simulink model "DCDC_Buck"  (R2021b)
settings: Solver=VariableStepAuto  StartTime=0.0  StopTime=10.0  RelTol=1e-3
model workspace (MAT data in the model file):
  VSF = 0.439
undefined symbols (not defined in the file): FPWM, Gi, TBPRD, Tpwm, Ts
libraries: fl_lib x24, nesl_utility x6, ee_lib x3, tiiqmathlib x2, simulink x2
settings Model: Creator=win  LastModifiedBy=win

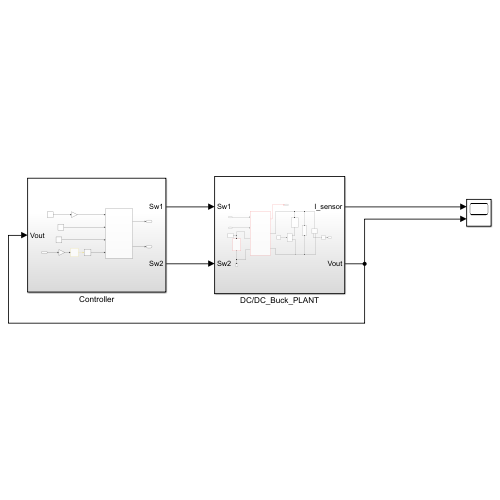
[thumbnail: Simulink's stored preview of the top-level diagram]
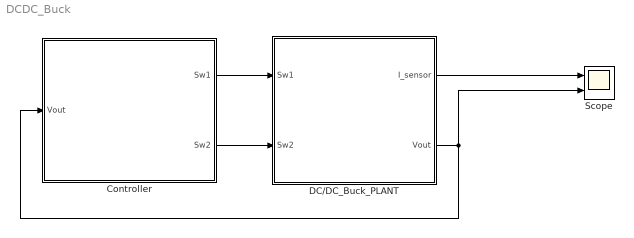
== system DCDC_Buck ==
  Controller : Subsystem
  DC/DC_Buck_PLANT : Subsystem
  Scope : Scope  NumInputPorts=2
  wires:
  Controller/1(Sw1) -> DC/DC_Buck_PLANT/1(Sw1)
  Controller/2(Sw2) -> DC/DC_Buck_PLANT/2(Sw2)
  DC/DC_Buck_PLANT/2(Vout) -> Controller/1(Vout), Scope/2
  DC/DC_Buck_PLANT/1(I_sensor) -> Scope/1

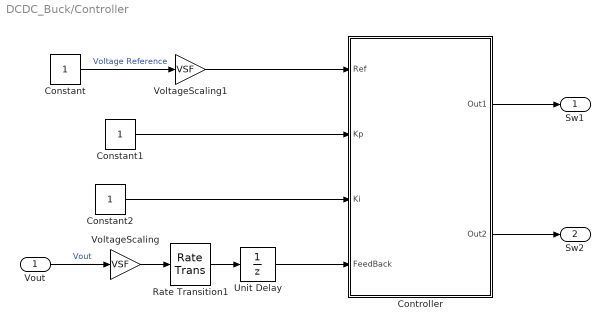
== system DCDC_Buck/Controller ==
  Vout : Inport
  Constant : Constant
  Constant1 : Constant
  Constant2 : Constant
  Controller : Subsystem
  Rate Transition1 : RateTransition  Integrity=off  Deterministic=off  OutPortSampleTime=Tcont
  Unit Delay : UnitDelay  SampleTime=-1  HasFrameUpgradeWarning=on
  VoltageScaling : Gain  Gain=VSF
  VoltageScaling1 : Gain  Gain=VSF
  Sw1 : Outport
  Sw2 : Outport  Port=2
  wires:
  Vout/1 -> VoltageScaling/1  "Vout"
  VoltageScaling/1 -> Rate Transition1/1
  Rate Transition1/1 -> Unit Delay/1
  Unit Delay/1 -> Controller/4(FeedBack)
  Constant/1 -> VoltageScaling1/1  "Voltage Reference"
  VoltageScaling1/1 -> Controller/1(Ref)
  Constant1/1 -> Controller/2(Kp)
  Constant2/1 -> Controller/3(Ki)
  Controller/1(Out1) -> Sw1/1
  Controller/2(Out2) -> Sw2/1

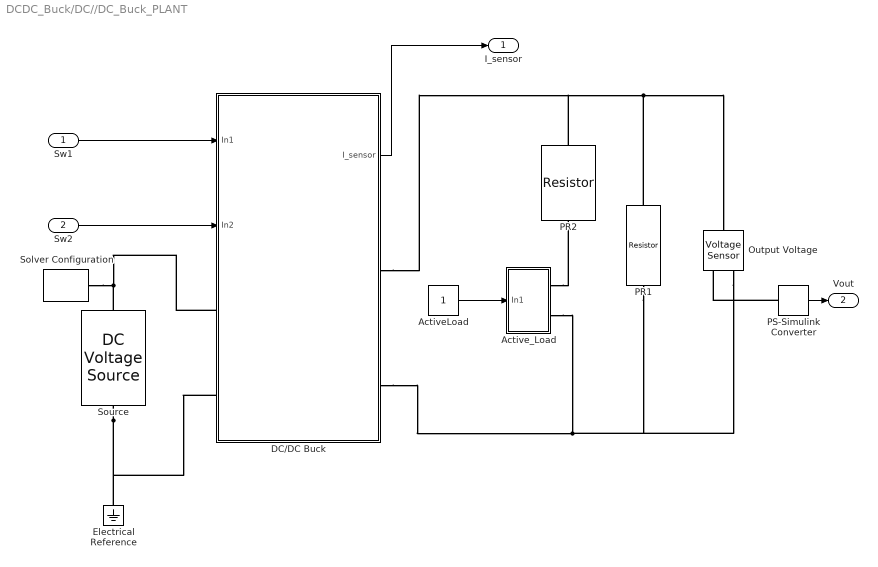
== system DCDC_Buck/DC//DC_Buck_PLANT ==
  Sw1 : Inport
  Sw2 : Inport  Port=2
  ActiveLoad : Constant
  Active_Load : Subsystem
  DC/DC Buck : Subsystem
  Electrical Reference : fl_lib/Electrical/Electrical Elements/Electrical Reference
  Output Voltage : fl_lib/Electrical/Electrical Sensors/Voltage Sensor  Priority=0
  PR1 : fl_lib/Electrical/Electrical Elements/Resistor  R=7.5 Ohm  i_specify=off  i_priority=None  i=0 A  i_nominal_specify=off  i_nominal_unit=A  i_nominal_value=1  v_specify=off  v_priority=None  v=0 V  v_nominal_specify=off  v_nominal_unit=V  v_nominal_value=1
  PR2 : fl_lib/Electrical/Electrical Elements/Resistor  R=2 Ohm  i_specify=off  i_priority=None  i=0 A  i_nominal_specify=off  i_nominal_unit=A  i_nominal_value=1  v_specify=off  v_priority=None  v=0 V  v_nominal_specify=off  v_nominal_unit=V  v_nominal_value=1
  PS-Simulink Converter : nesl_utility/PS-Simulink Converter  Priority=2  PhysicalDomain=network_engine_domain  SubClassName=ps_output  LeftPortType=input  RightPortType=output  PseudoPeriodic=off  Frequencies=[]  Unit=1  AffineConversion=off
      settings: SourceProductBaseCode=PW,SS
  Solver Configuration : nesl_utility/Solver Configuration  PhysicalDomain=network_engine_domain  SubClassName=solver  LeftPortType=input  RightPortType=generic  Tones=[]  Harmonics=[]  SimulateNoise=off  Profile=off  UseLocalSampling=off  EnableSwitchedLinearOptims=on  FrequencyDomain=off  UseCCode=off  RelTol=0.001  AbsTol=1e-06  MinStep=1e-09  ToWorkspace=off  RevertToSquareIcSolve=off  NumHomotopyIterations=100  PhasorMode=off  PhasorModeNumHarmonics=1  DoDC=off  ResidualTolerance=1e-08  UseLocalSolver=off  LocalSolverChoice=NE_TRAPEZOIDAL_ADVANCER  LocalSolverSampleTime=Ts/10  DoFixedCost=off  MaxNonlinIter=3  MaxModeIter=2  ComputeImpulses=off  ImpulseIterations=2  LinearAlgebra=Sparse  EquationFormulation=NE_TIME_EF  DelaysMemoryBudget=1024  AutomaticFiltering=on  FilteringTimeConstant=0.001  PartitionStorageMethod=AS_NEEDED  PartitionMemoryBudget=1024  PartitionMethod=FAST
      settings: SourceProductBaseCode=PW,SS
  Source : fl_lib/Electrical/Electrical Sources/DC Voltage Source  v0=9 V
  I_sensor : Outport  VectorParamsAs1DForOutWhenUnconnected=off
  Vout : Outport  Port=2  VectorParamsAs1DForOutWhenUnconnected=off
  wires:
  DC/DC Buck/1(I_sensor) -> I_sensor/1
  Sw2/1 -> DC/DC Buck/2(In2)
  Sw1/1 -> DC/DC Buck/1(In1)
  PS-Simulink Converter/1 -> Vout/1
  ActiveLoad/1 -> Active_Load/1(In1)
  connections:
  PS-Simulink Converter/LConn1 -- Output Voltage/RConn1
  Active_Load/RConn2 -- DC/DC Buck/RConn2 -- PR1/RConn1 -- Output Voltage/RConn2
  PR1/LConn1 -- Output Voltage/LConn1 -- DC/DC Buck/RConn1 -- PR2/LConn1
  Source/RConn1 -- DC/DC Buck/LConn2 -- Electrical Reference/LConn1
  Active_Load/RConn1 -- PR2/RConn1
  Solver Configuration/RConn1 -- DC/DC Buck/LConn1 -- Source/LConn1

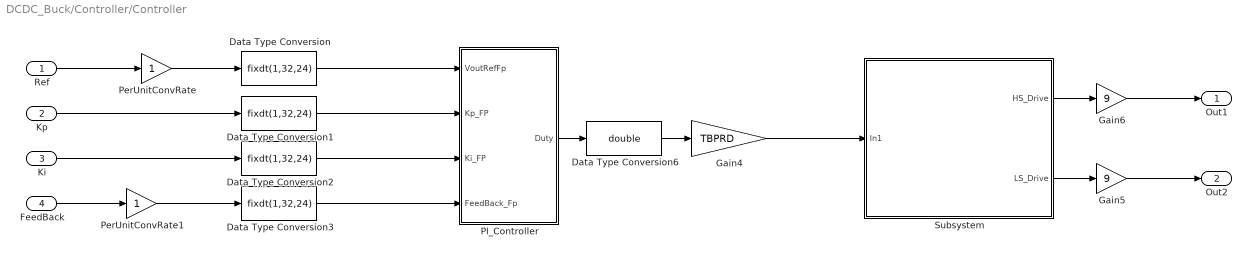
== system DCDC_Buck/Controller/Controller ==
  Ref : Inport
  Kp : Inport  Port=2
  Ki : Inport  Port=3
  FeedBack : Inport  Port=4
  Data Type Conversion{,1..3} (4 alike) : DataTypeConversion  OutDataTypeStr=fixdt(1,32,24)
  Data Type Conversion6 : DataTypeConversion  OutDataTypeStr=double
  Gain4 : Gain  Gain=TBPRD  ParamDataTypeStr=int16  OutDataTypeStr=fixdt(1,32,20)  RndMeth=Simplest
  Gain5 : Gain  Gain=9
  Gain6 : Gain  Gain=9
  PI_Controller : Subsystem
  PerUnitConvRate : Gain
  PerUnitConvRate1 : Gain
  Subsystem : Subsystem
  Out1 : Outport  VectorParamsAs1DForOutWhenUnconnected=off
  Out2 : Outport  Port=2  VectorParamsAs1DForOutWhenUnconnected=off
  wires:
  Ref/1 -> PerUnitConvRate/1
  PerUnitConvRate/1 -> Data Type Conversion/1
  Kp/1 -> Data Type Conversion1/1
  Ki/1 -> Data Type Conversion2/1
  FeedBack/1 -> PerUnitConvRate1/1
  PerUnitConvRate1/1 -> Data Type Conversion3/1
  Data Type Conversion/1 -> PI_Controller/1(VoutRefFp)
  Data Type Conversion1/1 -> PI_Controller/2(Kp_FP)
  Data Type Conversion2/1 -> PI_Controller/3(Ki_FP)
  Data Type Conversion3/1 -> PI_Controller/4(FeedBack_Fp)
  PI_Controller/1(Duty) -> Data Type Conversion6/1
  Data Type Conversion6/1 -> Gain4/1
  Gain4/1 -> Subsystem/1(In1)
  Subsystem/2(LS_Drive) -> Gain5/1
  Subsystem/1(HS_Drive) -> Gain6/1
  Gain6/1 -> Out1/1
  Gain5/1 -> Out2/1

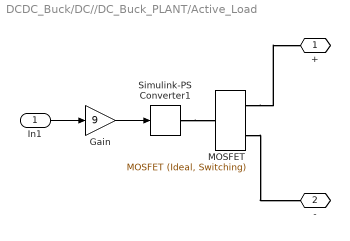
== system DCDC_Buck/DC//DC_Buck_PLANT/Active_Load ==
  In1 : Inport
  Gain : Gain  Gain=9
  MOSFET : ee_lib/Semiconductors & Converters/MOSFET (Ideal, Switching)  Rds=0.2 Ohm  Goff=1e-6 1/Ohm  Vth=3 V  diode_param=2  diode_Vf=1.6 V  diode_Ron=0.001 Ohm  diode_Goff=1e-5 1/Ohm  diode_C=5e-8 F  diode_iRM=-235 A  diode_iF=300 A  diode_idot=-100 A/us  diode_trr_param=2  diode_trr_factor=3  diode_trr=70 ns  diode_Qrr=1.5e+3 s*uA  thermal_loss_option=ee.enum.converters.thermalLossOption.constantvalues  Von_data=[0, 1.1, 1.3, 1.45, 1.75, 2.25, 2.7; 0, 1, 1.15, 1.35, 1.7, 2.35, 3] V  Tj=[298.15, 398.15] K  Iout_data=[0, 10, 50, 100, 200, 400, 600] A  Eon_data=[0, .29, 1.43, 2.86, 5.71, 13.14, 22.86; 0, .57, 2.63, 5.14, 10.29, 20.57, 30.29] * 1e-3 J  Eoff_data=[0, .21, 1.07, 2.14, 4.29, 9.86, 17.14; 0, .43, 1.97, 3.86, 7.71, 15.43, 22.71] * 1e-3 J  Tj_loss=[298.15, 398.15] K  Iout_data_loss=[0, 10, 50, 100, 200, 400, 600] A  Eon_scalar=22.86e-3 J  Eoff_scalar=17.14e-3 J  Voff=300 V  Iout_scalar=600 A  diodeModelType=ee.enum.converters.diodeModelType.pwl  diodeTableType=ee.enum.diode.tableType.IfMat  diode_IfMat=[.07, .12, .19, 1.75, 4.24, 7.32, 11.2; .16, .3, .72, 2.14, 4.02, 6.35, 9.12] A  diode_VfMat=[.9, 1.15, 1.25, 1.5, 1.75, 2.17, 2.6, 2.85; .58, .68, .75, 1.1, 1.38, 1.77, 2.27, 2.7] V  diode_TjVec=[25, 125] degC  diode_VfVec=[.5, .7, .9, 1.3, 1.7, 2.1, 2.5] V  diode_IfVec=[.1, .2, .5, 1, 2, 4, 7, 10] A  diode_Vr=-600 V  diode_Ls=150 nH  diode_Erec=0.03 J  thermal_network_parameterization=ee.enum.thermalNetworkTopology.external  Rth=[.03, .2] K/W  Rth_Cauer=[.03, .1, .2] K/W  Rth_Foster=[.03, .2] K/W  thermal_mass_parameterization=ee.enum.thermalNetwork.timeconstant  thermal_mass=[3, 25] J/K  thermal_mass_Cauer=[3, 10, 25] J/K  thermal_mass_Foster=[33, 50] J/K  thermal_time_constant=[.1, 5] s  thermal_time_constant_Cauer=[.1, 1, 5] s  thermal_time_constant_Foster=[1, 10] s  thermal_mass_initial_temperatures=[25, 25] degC  thermal_mass_initial_temperatures_Cauer=[25, 25, 25] degC  junction_thermal_mass=0.1 J/K  steadyState_Foster=simscape.enum.onoff.on  Tvec_initial_Foster=[25, 25, 25, 25] degC  no_thermal_network=0  junction_temperature_specify=off  junction_temperature_priority=None  junction_temperature=25 degC  junction_temperature_nominal_specify=off  junction_temperature_nominal_unit=degC  junction_temperature_nominal_value=1  vT_specify=off  vT_priority=None  vT=0 V  vT_nominal_specify=off  vT_nominal_unit=V  vT_nominal_value=1  Qj_specify=off  Qj_priority=None  Qj=0 W  Qj_nominal_specify=off  Qj_nominal_unit=W  Qj_nominal_value=1
  Simulink-PS Converter1 : nesl_utility/Simulink-PS Converter  PhysicalDomain=network_engine_domain  SubClassName=ps_input  LeftPortType=input  RightPortType=output  PseudoPeriodic=off  Frequencies=[]  NoiseDistribution=none  NoiseParameters=[]  Unit=1  AffineConversion=off  FilteringAndDerivatives=provide  SimscapeFilterOrder=1  InputFilterTimeConstant=0.001  UdotUserProvided=0
      settings: SourceProductBaseCode=PW,SS
  + : PMIOPort  Side=Right
  - : PMIOPort  Port=2  Side=Right
  wires:
  Gain/1 -> Simulink-PS Converter1/1
  In1/1 -> Gain/1
  connections:
  Simulink-PS Converter1/RConn1 -- MOSFET/LConn1
  MOSFET/RConn1 -- +/RConn1
  MOSFET/RConn2 -- -/RConn1

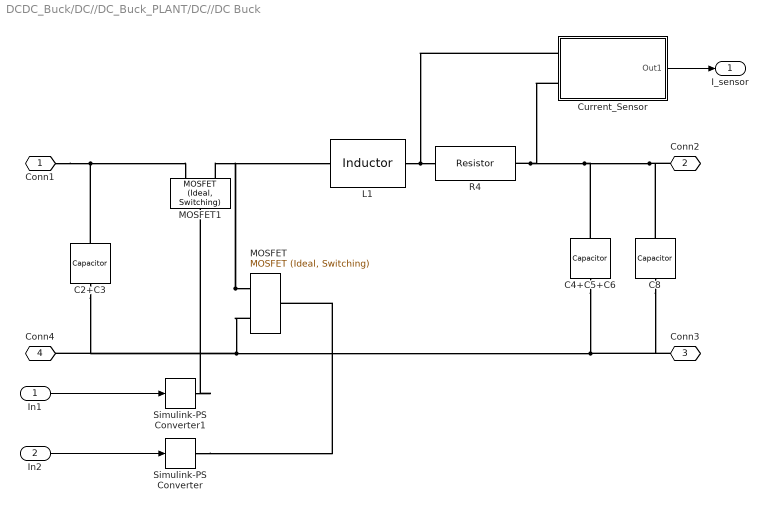
== system DCDC_Buck/DC//DC_Buck_PLANT/DC//DC Buck ==
  In1 : Inport
  In2 : Inport  Port=2
  C2+C3 : fl_lib/Electrical/Electrical Elements/Capacitor  c=44 uF  r=1e-6 Ohm  g=0 1/Ohm  i_specify=off  i_priority=None  i=0 A  i_nominal_specify=off  i_nominal_unit=A  i_nominal_value=1  v_specify=off  v_priority=None  v=0 V  v_nominal_specify=off  v_nominal_unit=V  v_nominal_value=1  vc_specify=off  vc_priority=High  vc=0 V  vc_nominal_specify=off  vc_nominal_unit=V  vc_nominal_value=1
  C4+C5+C6 : fl_lib/Electrical/Electrical Elements/Capacitor  c=66 uF  r=0.002 Ohm  g=0 1/Ohm  i_specify=off  i_priority=None  i=0 A  i_nominal_specify=off  i_nominal_unit=A  i_nominal_value=1  v_specify=off  v_priority=None  v=0 V  v_nominal_specify=off  v_nominal_unit=V  v_nominal_value=1  vc_specify=off  vc_priority=High  vc=0 V  vc_nominal_specify=off  vc_nominal_unit=V  vc_nominal_value=1
  C8 : fl_lib/Electrical/Electrical Elements/Capacitor  c=330 uF  r=0.002 Ohm  g=0 1/Ohm  i_specify=off  i_priority=None  i=0 A  i_nominal_specify=off  i_nominal_unit=A  i_nominal_value=1  v_specify=off  v_priority=None  v=0 V  v_nominal_specify=off  v_nominal_unit=V  v_nominal_value=1  vc_specify=off  vc_priority=High  vc=0 V  vc_nominal_specify=off  vc_nominal_unit=V  vc_nominal_value=1
  Current_Sensor : Subsystem
  L1 : fl_lib/Electrical/Electrical Elements/Inductor  l=4.8 uH  r=0.0105 Ohm  g=0 1/Ohm  i_specify=off  i_priority=None  i=0 A  i_nominal_specify=off  i_nominal_unit=A  i_nominal_value=1  v_specify=off  v_priority=None  v=0 V  v_nominal_specify=off  v_nominal_unit=V  v_nominal_value=1  i_L_specify=off  i_L_priority=High  i_L=0 A  i_L_nominal_specify=off  i_L_nominal_unit=A  i_L_nominal_value=1
  MOSFET : ee_lib/Semiconductors & Converters/MOSFET (Ideal, Switching)  Rds=3e-3 Ohm  Goff=1e-6 1/Ohm  Vth=1.5 V  diode_param=2  diode_Vf=0.78 V  diode_Ron=0.001 Ohm  diode_Goff=1e-5 1/Ohm  diode_C=5e-8 F  diode_iRM=-235 A  diode_iF=300 A  diode_idot=-50 A/us  diode_trr_param=1  diode_trr_factor=3  diode_trr=15 us  diode_Qrr=1.5e+3 s*uA  thermal_loss_option=ee.enum.converters.thermalLossOption.constantvalues  Von_data=[0, 1.1, 1.3, 1.45, 1.75, 2.25, 2.7; 0, 1, 1.15, 1.35, 1.7, 2.35, 3] V  Tj=[298.15, 398.15] K  Iout_data=[0, 10, 50, 100, 200, 400, 600] A  Eon_data=[0, .29, 1.43, 2.86, 5.71, 13.14, 22.86; 0, .57, 2.63, 5.14, 10.29, 20.57, 30.29] * 1e-3 J  Eoff_data=[0, .21, 1.07, 2.14, 4.29, 9.86, 17.14; 0, .43, 1.97, 3.86, 7.71, 15.43, 22.71] * 1e-3 J  Tj_loss=[298.15, 398.15] K  Iout_data_loss=[0, 10, 50, 100, 200, 400, 600] A  Eon_scalar=22.86e-3 J  Eoff_scalar=17.14e-3 J  Voff=300 V  Iout_scalar=600 A  diodeModelType=ee.enum.converters.diodeModelType.pwl  diodeTableType=ee.enum.diode.tableType.IfMat  diode_IfMat=[.07, .12, .19, 1.75, 4.24, 7.32, 11.2; .16, .3, .72, 2.14, 4.02, 6.35, 9.12] A  diode_VfMat=[.9, 1.15, 1.25, 1.5, 1.75, 2.17, 2.6, 2.85; .58, .68, .75, 1.1, 1.38, 1.77, 2.27, 2.7] V  diode_TjVec=[25, 125] degC  diode_VfVec=[.5, .7, .9, 1.3, 1.7, 2.1, 2.5] V  diode_IfVec=[.1, .2, .5, 1, 2, 4, 7, 10] A  diode_Vr=-600 V  diode_Ls=150 nH  diode_Erec=0.03 J  thermal_network_parameterization=ee.enum.thermalNetworkTopology.external  Rth=[.03, .2] K/W  Rth_Cauer=[.03, .1, .2] K/W  Rth_Foster=[.03, .2] K/W  thermal_mass_parameterization=ee.enum.thermalNetwork.timeconstant  thermal_mass=[3, 25] J/K  thermal_mass_Cauer=[3, 10, 25] J/K  thermal_mass_Foster=[33, 50] J/K  thermal_time_constant=[.1, 5] s  thermal_time_constant_Cauer=[.1, 1, 5] s  thermal_time_constant_Foster=[1, 10] s  thermal_mass_initial_temperatures=[25, 25] degC  thermal_mass_initial_temperatures_Cauer=[25, 25, 25] degC  junction_thermal_mass=0.1 J/K  steadyState_Foster=simscape.enum.onoff.on  Tvec_initial_Foster=[25, 25, 25, 25] degC  no_thermal_network=0  junction_temperature_specify=off  junction_temperature_priority=None  junction_temperature=25 degC  junction_temperature_nominal_specify=off  junction_temperature_nominal_unit=degC  junction_temperature_nominal_value=1  vT_specify=off  vT_priority=None  vT=0 V  vT_nominal_specify=off  vT_nominal_unit=V  vT_nominal_value=1  Qj_specify=off  Qj_priority=None  Qj=0 W  Qj_nominal_specify=off  Qj_nominal_unit=W  Qj_nominal_value=1
  MOSFET1 : ee_lib/Semiconductors & Converters/MOSFET (Ideal, Switching)  Rds=9e-3 Ohm  Goff=1e-6 1/Ohm  Vth=1.5 V  diode_param=2  diode_Vf=0.85 V  diode_Ron=0.001 Ohm  diode_Goff=1e-5 1/Ohm  diode_C=5e-8 F  diode_iRM=-235 A  diode_iF=300 A  diode_idot=-50 A/us  diode_trr_param=3  diode_trr_factor=3  diode_trr=15 us  diode_Qrr=1.5e+3 s*uA  thermal_loss_option=ee.enum.converters.thermalLossOption.constantvalues  Von_data=[0, 1.1, 1.3, 1.45, 1.75, 2.25, 2.7; 0, 1, 1.15, 1.35, 1.7, 2.35, 3] V  Tj=[298.15, 398.15] K  Iout_data=[0, 10, 50, 100, 200, 400, 600] A  Eon_data=[0, .29, 1.43, 2.86, 5.71, 13.14, 22.86; 0, .57, 2.63, 5.14, 10.29, 20.57, 30.29] * 1e-3 J  Eoff_data=[0, .21, 1.07, 2.14, 4.29, 9.86, 17.14; 0, .43, 1.97, 3.86, 7.71, 15.43, 22.71] * 1e-3 J  Tj_loss=[298.15, 398.15] K  Iout_data_loss=[0, 10, 50, 100, 200, 400, 600] A  Eon_scalar=22.86e-3 J  Eoff_scalar=17.14e-3 J  Voff=300 V  Iout_scalar=600 A  diodeModelType=ee.enum.converters.diodeModelType.pwl  diodeTableType=ee.enum.diode.tableType.IfMat  diode_IfMat=[.07, .12, .19, 1.75, 4.24, 7.32, 11.2; .16, .3, .72, 2.14, 4.02, 6.35, 9.12] A  diode_VfMat=[.9, 1.15, 1.25, 1.5, 1.75, 2.17, 2.6, 2.85; .58, .68, .75, 1.1, 1.38, 1.77, 2.27, 2.7] V  diode_TjVec=[25, 125] degC  diode_VfVec=[.5, .7, .9, 1.3, 1.7, 2.1, 2.5] V  diode_IfVec=[.1, .2, .5, 1, 2, 4, 7, 10] A  diode_Vr=-600 V  diode_Ls=150 nH  diode_Erec=0.03 J  thermal_network_parameterization=ee.enum.thermalNetworkTopology.external  Rth=[.03, .2] K/W  Rth_Cauer=[.03, .1, .2] K/W  Rth_Foster=[.03, .2] K/W  thermal_mass_parameterization=ee.enum.thermalNetwork.timeconstant  thermal_mass=[3, 25] J/K  thermal_mass_Cauer=[3, 10, 25] J/K  thermal_mass_Foster=[33, 50] J/K  thermal_time_constant=[.1, 5] s  thermal_time_constant_Cauer=[.1, 1, 5] s  thermal_time_constant_Foster=[1, 10] s  thermal_mass_initial_temperatures=[25, 25] degC  thermal_mass_initial_temperatures_Cauer=[25, 25, 25] degC  junction_thermal_mass=0.1 J/K  steadyState_Foster=simscape.enum.onoff.on  Tvec_initial_Foster=[25, 25, 25, 25] degC  no_thermal_network=0  junction_temperature_specify=off  junction_temperature_priority=None  junction_temperature=25 degC  junction_temperature_nominal_specify=off  junction_temperature_nominal_unit=degC  junction_temperature_nominal_value=1  vT_specify=off  vT_priority=None  vT=0 V  vT_nominal_specify=off  vT_nominal_unit=V  vT_nominal_value=1  Qj_specify=off  Qj_priority=None  Qj=0 W  Qj_nominal_specify=off  Qj_nominal_unit=W  Qj_nominal_value=1
  R4 : fl_lib/Electrical/Electrical Elements/Resistor  R=0.03 Ohm  i_specify=off  i_priority=None  i=0 A  i_nominal_specify=off  i_nominal_unit=A  i_nominal_value=1  v_specify=off  v_priority=None  v=0 V  v_nominal_specify=off  v_nominal_unit=V  v_nominal_value=1
  Simulink-PS Converter : nesl_utility/Simulink-PS Converter  PhysicalDomain=network_engine_domain  SubClassName=ps_input  LeftPortType=input  RightPortType=output  PseudoPeriodic=off  Frequencies=[]  NoiseDistribution=none  NoiseParameters=[]  Unit=1  AffineConversion=off  FilteringAndDerivatives=provide  SimscapeFilterOrder=1  InputFilterTimeConstant=0.001  UdotUserProvided=0
      settings: SourceProductBaseCode=PW,SS
  Simulink-PS Converter1 : nesl_utility/Simulink-PS Converter  PhysicalDomain=network_engine_domain  SubClassName=ps_input  LeftPortType=input  RightPortType=output  PseudoPeriodic=off  Frequencies=[]  NoiseDistribution=none  NoiseParameters=[]  Unit=1  AffineConversion=off  FilteringAndDerivatives=provide  SimscapeFilterOrder=1  InputFilterTimeConstant=0.001  UdotUserProvided=0
      settings: SourceProductBaseCode=PW,SS
  Conn1 : PMIOPort  Side=Left
  Conn2 : PMIOPort  Port=2  Side=Right
  Conn3 : PMIOPort  Port=3  Side=Right
  Conn4 : PMIOPort  Port=4  Side=Left
  I_sensor : Outport  VectorParamsAs1DForOutWhenUnconnected=off
  wires:
  Current_Sensor/1(Out1) -> I_sensor/1
  In2/1 -> Simulink-PS Converter/1
  In1/1 -> Simulink-PS Converter1/1
  connections:
  R4/RConn1 -- C4+C5+C6/LConn1 -- C8/LConn1 -- Conn2/RConn1 -- Current_Sensor/LConn2
  MOSFET/RConn1 -- L1/LConn1 -- MOSFET1/RConn2
  Simulink-PS Converter/RConn1 -- MOSFET/LConn1
  Simulink-PS Converter1/RConn1 -- MOSFET1/LConn1
  Conn1/RConn1 -- C2+C3/LConn1 -- MOSFET1/RConn1
  R4/LConn1 -- Current_Sensor/LConn1 -- L1/RConn1
  C4+C5+C6/RConn1 -- C8/RConn1 -- Conn3/RConn1 -- MOSFET/RConn2 -- C2+C3/RConn1 -- Conn4/RConn1

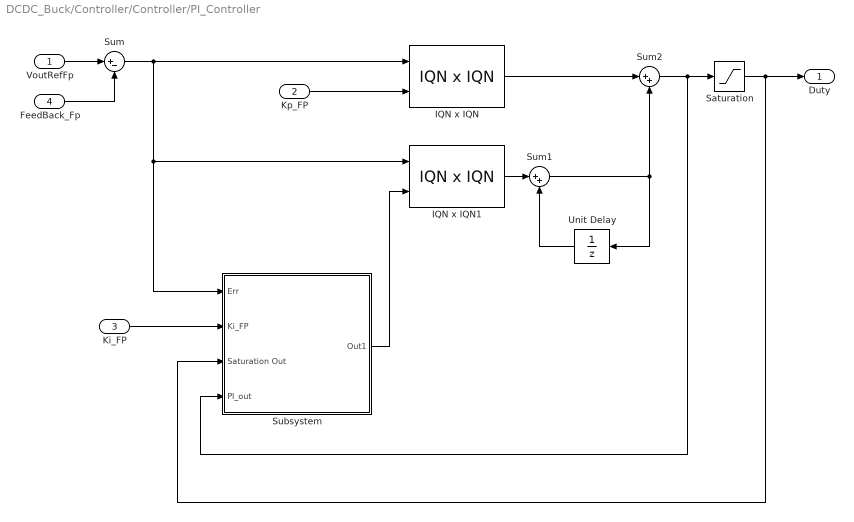
== system DCDC_Buck/Controller/Controller/PI_Controller ==
  VoutRefFp : Inport
  Kp_FP : Inport  Port=2
  Ki_FP : Inport  Port=3
  FeedBack_Fp : Inport  Port=4
  IQN x IQN : tiiqmathlib/IQN x IQN  multiplyOption=Multiply
      settings: SourceProductBaseCode=TIC2000
  IQN x IQN1 : tiiqmathlib/IQN x IQN  multiplyOption=Multiply
      settings: SourceProductBaseCode=TIC2000
  Saturation : Saturate  UpperLimit=0.8  LowerLimit=0
  Subsystem : Subsystem
  Sum : Sum  Inputs=|+-
  Sum1 : Sum  Inputs=|++
  Sum2 : Sum  Inputs=|++
  Unit Delay : UnitDelay  SampleTime=-1  HasFrameUpgradeWarning=on
  Duty : Outport
  wires:
  VoutRefFp/1 -> Sum/1
  FeedBack_Fp/1 -> Sum/2
  Sum/1 -> Subsystem/1(Err), IQN x IQN1/1, IQN x IQN/1
  Kp_FP/1 -> IQN x IQN/2
  IQN x IQN1/1 -> Sum1/1
  Sum1/1 -> Unit Delay/1, Sum2/2
  Unit Delay/1 -> Sum1/2
  IQN x IQN/1 -> Sum2/1
  Sum2/1 -> Subsystem/4(PI_out), Saturation/1
  Saturation/1 -> Subsystem/3(Saturation Out), Duty/1
  Subsystem/1(Out1) -> IQN x IQN1/2
  Ki_FP/1 -> Subsystem/2(Ki_FP)

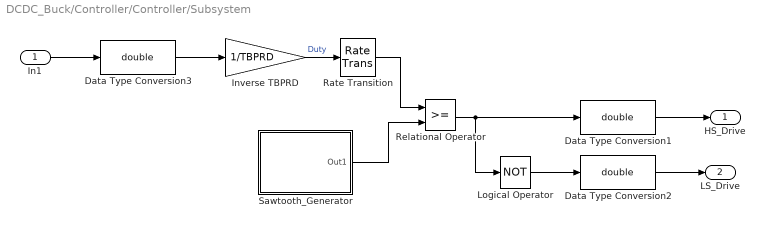
== system DCDC_Buck/Controller/Controller/Subsystem ==
  In1 : Inport
  Data Type Conversion1 : DataTypeConversion  OutDataTypeStr=double
  Data Type Conversion2 : DataTypeConversion  OutDataTypeStr=double
  Data Type Conversion3 : DataTypeConversion  OutDataTypeStr=double
  Inverse TBPRD : Gain  Gain=1/TBPRD  RndMeth=Simplest
  Logical Operator : Logic  Operator=NOT  AllPortsSameDT=off  OutDataTypeStr=boolean
  Rate Transition : RateTransition  OutPortSampleTime=0
      settings: AttributesFormatString=Ts = %<OutPortSampleTime>
  Relational Operator : RelationalOperator  OutDataTypeStr=boolean  RndMeth=Simplest
  Sawtooth_Generator : Subsystem
  HS_Drive : Outport
  LS_Drive : Outport  Port=2
  wires:
  In1/1 -> Data Type Conversion3/1
  Data Type Conversion3/1 -> Inverse TBPRD/1
  Inverse TBPRD/1 -> Rate Transition/1  "Duty"
  Rate Transition/1 -> Relational Operator/1
  Sawtooth_Generator/1(Out1) -> Relational Operator/2
  Data Type Conversion1/1 -> HS_Drive/1
  Relational Operator/1 -> Logical Operator/1, Data Type Conversion1/1
  Logical Operator/1 -> Data Type Conversion2/1
  Data Type Conversion2/1 -> LS_Drive/1

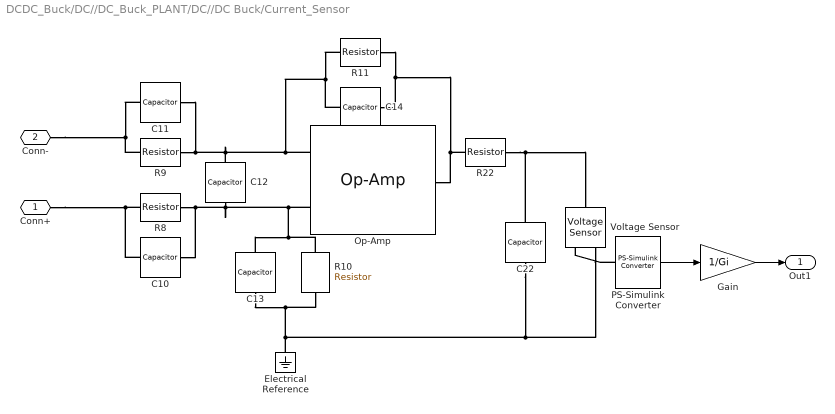
== system DCDC_Buck/DC//DC_Buck_PLANT/DC//DC Buck/Current_Sensor ==
  C10 : fl_lib/Electrical/Electrical Elements/Capacitor  c=220 pF  r=1e-6 Ohm  g=0 1/Ohm  i_specify=off  i_priority=None  i=0 A  i_nominal_specify=off  i_nominal_unit=A  i_nominal_value=1  v_specify=off  v_priority=None  v=0 V  v_nominal_specify=off  v_nominal_unit=V  v_nominal_value=1  vc_specify=off  vc_priority=High  vc=0 V  vc_nominal_specify=off  vc_nominal_unit=V  vc_nominal_value=1
  C11 : fl_lib/Electrical/Electrical Elements/Capacitor  c=220 pF  r=1e-6 Ohm  g=0 1/Ohm  i_specify=off  i_priority=None  i=0 A  i_nominal_specify=off  i_nominal_unit=A  i_nominal_value=1  v_specify=off  v_priority=None  v=0 V  v_nominal_specify=off  v_nominal_unit=V  v_nominal_value=1  vc_specify=off  vc_priority=High  vc=0 V  vc_nominal_specify=off  vc_nominal_unit=V  vc_nominal_value=1
  C12 : fl_lib/Electrical/Electrical Elements/Capacitor  c=1 nF  r=1e-6 Ohm  g=0 1/Ohm  i_specify=off  i_priority=None  i=0 A  i_nominal_specify=off  i_nominal_unit=A  i_nominal_value=1  v_specify=off  v_priority=None  v=0 V  v_nominal_specify=off  v_nominal_unit=V  v_nominal_value=1  vc_specify=off  vc_priority=High  vc=0 V  vc_nominal_specify=off  vc_nominal_unit=V  vc_nominal_value=1
  C13 : fl_lib/Electrical/Electrical Elements/Capacitor  c=10 pF  r=1e-6 Ohm  g=0 1/Ohm  i_specify=off  i_priority=None  i=0 A  i_nominal_specify=off  i_nominal_unit=A  i_nominal_value=1  v_specify=off  v_priority=None  v=0 V  v_nominal_specify=off  v_nominal_unit=V  v_nominal_value=1  vc_specify=off  vc_priority=High  vc=0 V  vc_nominal_specify=off  vc_nominal_unit=V  vc_nominal_value=1
  C14 : fl_lib/Electrical/Electrical Elements/Capacitor  c=10 pF  r=1e-6 Ohm  g=0 1/Ohm  i_specify=off  i_priority=None  i=0 A  i_nominal_specify=off  i_nominal_unit=A  i_nominal_value=1  v_specify=off  v_priority=None  v=0 V  v_nominal_specify=off  v_nominal_unit=V  v_nominal_value=1  vc_specify=off  vc_priority=High  vc=0 V  vc_nominal_specify=off  vc_nominal_unit=V  vc_nominal_value=1
  C22 : fl_lib/Electrical/Electrical Elements/Capacitor  c=3.3 nF  r=1e-6 Ohm  g=0 1/Ohm  i_specify=off  i_priority=None  i=0 A  i_nominal_specify=off  i_nominal_unit=A  i_nominal_value=1  v_specify=off  v_priority=None  v=0 V  v_nominal_specify=off  v_nominal_unit=V  v_nominal_value=1  vc_specify=off  vc_priority=High  vc=0 V  vc_nominal_specify=off  vc_nominal_unit=V  vc_nominal_value=1
  Electrical Reference : fl_lib/Electrical/Electrical Elements/Electrical Reference
  Gain : Gain  Gain=1/Gi
  Op-Amp : fl_lib/Electrical/Electrical Elements/Op-Amp  outI_specify=off  outI_priority=None  outI=0 A  outI_nominal_specify=off  outI_nominal_unit=A  outI_nominal_value=1
  PS-Simulink Converter : nesl_utility/PS-Simulink Converter  PhysicalDomain=network_engine_domain  SubClassName=ps_output  LeftPortType=input  RightPortType=output  PseudoPeriodic=off  Frequencies=[]  Unit=1  AffineConversion=off
      settings: SourceProductBaseCode=PW,SS
  R10 : fl_lib/Electrical/Electrical Elements/Resistor  R=1.2 kOhm  i_specify=off  i_priority=None  i=0 A  i_nominal_specify=off  i_nominal_unit=A  i_nominal_value=1  v_specify=off  v_priority=None  v=0 V  v_nominal_specify=off  v_nominal_unit=V  v_nominal_value=1
  R11 : fl_lib/Electrical/Electrical Elements/Resistor  R=1.2 kOhm  i_specify=off  i_priority=None  i=0 A  i_nominal_specify=off  i_nominal_unit=A  i_nominal_value=1  v_specify=off  v_priority=None  v=0 V  v_nominal_specify=off  v_nominal_unit=V  v_nominal_value=1
  R22 : fl_lib/Electrical/Electrical Elements/Resistor  R=1 kOhm  i_specify=off  i_priority=None  i=0 A  i_nominal_specify=off  i_nominal_unit=A  i_nominal_value=1  v_specify=off  v_priority=None  v=0 V  v_nominal_specify=off  v_nominal_unit=V  v_nominal_value=1
  R8 : fl_lib/Electrical/Electrical Elements/Resistor  R=82 Ohm  i_specify=off  i_priority=None  i=0 A  i_nominal_specify=off  i_nominal_unit=A  i_nominal_value=1  v_specify=off  v_priority=None  v=0 V  v_nominal_specify=off  v_nominal_unit=V  v_nominal_value=1
  R9 : fl_lib/Electrical/Electrical Elements/Resistor  R=82 Ohm  i_specify=off  i_priority=None  i=0 A  i_nominal_specify=off  i_nominal_unit=A  i_nominal_value=1  v_specify=off  v_priority=None  v=0 V  v_nominal_specify=off  v_nominal_unit=V  v_nominal_value=1
  Voltage Sensor : fl_lib/Electrical/Electrical Sensors/Voltage Sensor
  Conn+ : PMIOPort  Side=Left
  Conn- : PMIOPort  Port=2  Side=Left
  Out1 : Outport  VectorParamsAs1DForOutWhenUnconnected=off
  wires:
  Gain/1 -> Out1/1
  PS-Simulink Converter/1 -> Gain/1
  connections:
  C22/LConn1 -- R22/RConn1 -- Voltage Sensor/LConn1
  Op-Amp/RConn1 -- R22/LConn1 -- C14/RConn1 -- R11/RConn1
  C13/RConn1 -- R10/RConn1 -- Voltage Sensor/RConn2 -- C22/RConn1 -- Electrical Reference/LConn1
  C10/LConn1 -- R8/LConn1 -- Conn+/RConn1
  C11/LConn1 -- R9/LConn1 -- Conn-/RConn1
  C11/RConn1 -- R9/RConn1 -- C12/LConn1 -- Op-Amp/LConn2 -- C14/LConn1 -- R11/LConn1
  PS-Simulink Converter/LConn1 -- Voltage Sensor/RConn1
  C10/RConn1 -- R8/RConn1 -- C12/RConn1 -- C13/LConn1 -- R10/LConn1 -- Op-Amp/LConn1

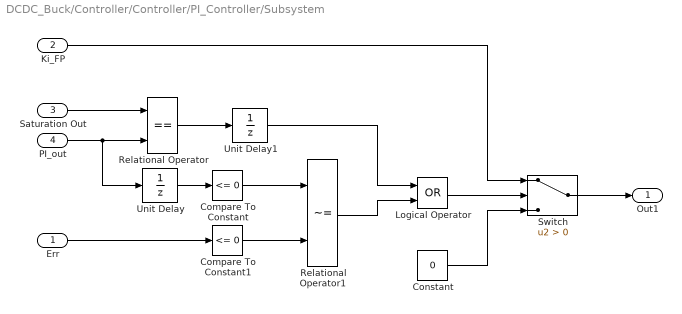
== system DCDC_Buck/Controller/Controller/PI_Controller/Subsystem ==
  Err : Inport
  Ki_FP : Inport  Port=2
  Saturation Out : Inport  Port=3
  PI_out : Inport  Port=4
  Compare To Constant : simulink/Logic and Bit Operations/Compare To Constant  relop=<=  const=0  OutDataTypeStr=boolean
  Compare To Constant1 : simulink/Logic and Bit Operations/Compare To Constant  relop=<=  const=0  OutDataTypeStr=boolean
  Constant : Constant  Value=0
  Logical Operator : Logic  Operator=OR  AllPortsSameDT=off  OutDataTypeStr=boolean
  Relational Operator : RelationalOperator  Operator===  OutDataTypeStr=boolean  RndMeth=Simplest
  Relational Operator1 : RelationalOperator  Operator=~=  OutDataTypeStr=boolean  RndMeth=Simplest
  Switch : Switch  Criteria=u2 > Threshold
  Unit Delay : UnitDelay  SampleTime=-1  HasFrameUpgradeWarning=on
  Unit Delay1 : UnitDelay  SampleTime=-1  HasFrameUpgradeWarning=on
  Out1 : Outport
  wires:
  PI_out/1 -> Unit Delay/1, Relational Operator/2
  Saturation Out/1 -> Relational Operator/1
  Unit Delay/1 -> Compare To Constant/1
  Compare To Constant/1 -> Relational Operator1/1
  Relational Operator/1 -> Unit Delay1/1
  Unit Delay1/1 -> Logical Operator/1
  Relational Operator1/1 -> Logical Operator/2
  Err/1 -> Compare To Constant1/1
  Compare To Constant1/1 -> Relational Operator1/2
  Logical Operator/1 -> Switch/2
  Ki_FP/1 -> Switch/1
  Constant/1 -> Switch/3
  Switch/1 -> Out1/1

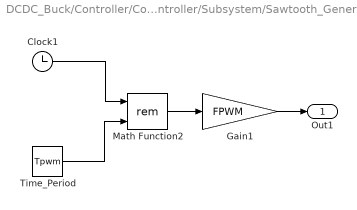
== system DCDC_Buck/Controller/Controller/Subsystem/Sawtooth_Generator ==
  Clock1 : Clock
  Gain1 : Gain  Gain=FPWM
  Math Function2 : Math  Operator=rem  SignedPower=on  SaturateOnIntegerOverflow=on
  Time_Period : Constant  Value=Tpwm
  Out1 : Outport  VectorParamsAs1DForOutWhenUnconnected=off
  wires:
  Gain1/1 -> Out1/1
  Math Function2/1 -> Gain1/1
  Time_Period/1 -> Math Function2/2
  Clock1/1 -> Math Function2/1
